simulink model "atmoDrag_test"  (R2018b)
settings: Solver=VariableStepAuto  StartTime=0.0  StopTime=10.0  RelTol=1e-3
undefined symbols (not defined in the file): simParams
libraries: atmoDrag_lib x1, clock_lib x1, time_Lib x1
settings Model: Creator=Taylor  LastModifiedBy=Taylor

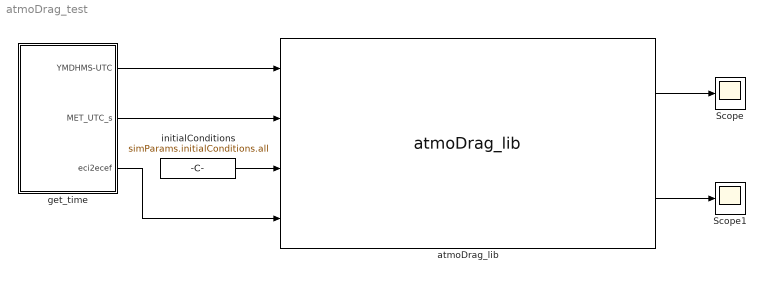
== system atmoDrag_test ==
  Scope : Scope
  Scope1 : Scope
  atmoDrag_lib : atmoDrag_lib/atmoDrag_lib  SystemSampleTime=-1
  get_time : Subsystem
  initialConditions : Constant  Value=simParams.initialConditions.all
  wires:
  get_time/1(YMDHMS-UTC) -> atmoDrag_lib/1
  get_time/3(eci2ecef) -> atmoDrag_lib/4
  get_time/2(MET_UTC_s) -> atmoDrag_lib/2
  initialConditions/1 -> atmoDrag_lib/3
  atmoDrag_lib/1 -> Scope/1
  atmoDrag_lib/2 -> Scope1/1

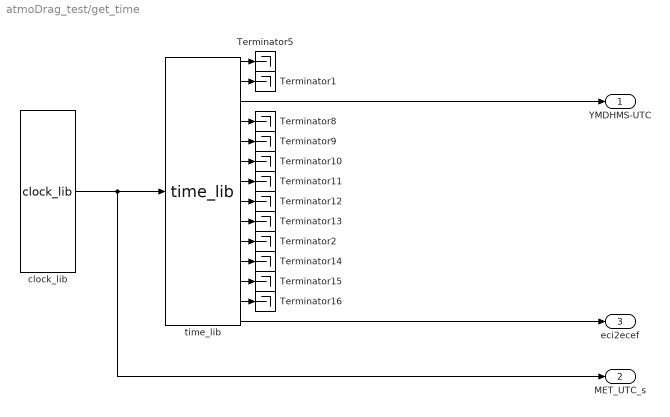
== system atmoDrag_test/get_time ==
  Terminator{1..2,5,8..16} (12 alike) : Terminator
  clock_lib : clock_lib/clock_lib  SystemSampleTime=-1
  "time_lib " : time_Lib/time_lib    SystemSampleTime=-1
  YMDHMS-UTC : Outport
  MET_UTC_s : Outport  Port=2
  eci2ecef : Outport  Port=3
  wires:
  "time_lib "/3 -> YMDHMS-UTC/1
  "time_lib "/14 -> eci2ecef/1
  "time_lib "/11 -> Terminator14/1
  "time_lib "/2 -> Terminator1/1
  "time_lib "/13 -> Terminator16/1
  "time_lib "/7 -> Terminator11/1
  "time_lib "/1 -> Terminator5/1
  "time_lib "/12 -> Terminator15/1
  "time_lib "/5 -> Terminator9/1
  "time_lib "/8 -> Terminator12/1
  "time_lib "/4 -> Terminator8/1
  "time_lib "/10 -> Terminator2/1
  clock_lib/1 -> MET_UTC_s/1, "time_lib "/1
  "time_lib "/9 -> Terminator13/1
  "time_lib "/6 -> Terminator10/1
